simulink model "trng_controller_emu"  (R2024a)
settings: Solver=FixedStepAuto  StartTime=0.0  StopTime=250  FixedStep=20e-3  RelTol=1e-3
model workspace (MAT data in the model file):
  Ki = 10
  Kp = 100
undefined symbols (not defined in the file or in its folder): DiscIntNeverNeededParam
libraries: dspstat3 x3
settings Model: Creator=manik  LastModifiedBy=manik

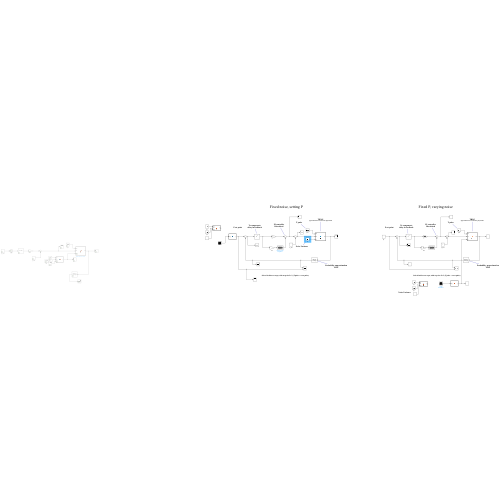
[thumbnail: Simulink's stored preview of the top-level diagram]
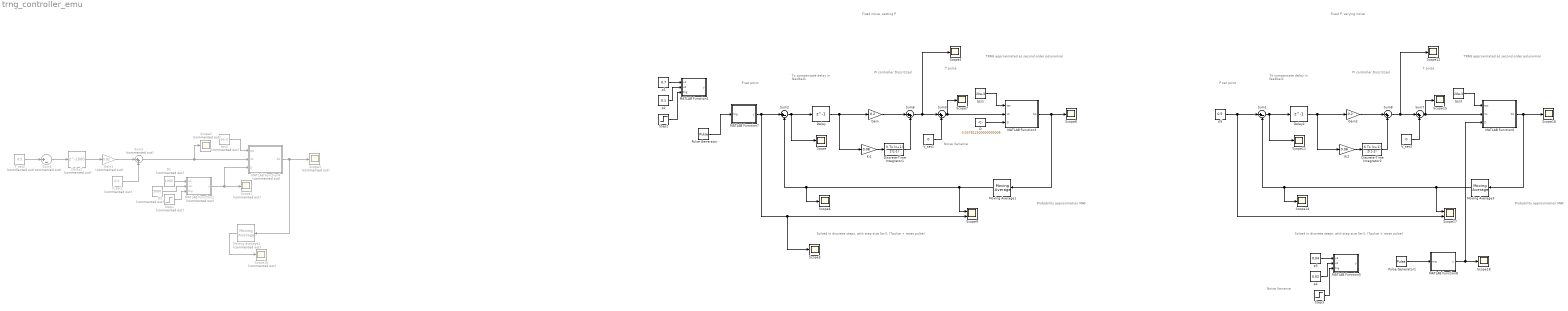
== system trng_controller_emu ==
  note: Fixed P, varying noise
  note: To compensate
      | delay in feedback
  note: PI controller
      | Discritized
  note: TRNG
      | approximated as second order polynomial
  note: T pulse
  note: Noise Variance
  note: Probability approximation
      | MAF
  note: Solved in discrete steps, with step size 5e-3, (Tpulse + reset pulse)
  note: P set point
  note: To compensate
      | delay in feedback
  note: PI controller
      | Discritized
  note: T pulse
  note: Probability approximation
      | MAF
  note: TRNG
      | approximated as second order polynomial
  note: Solved in discrete steps, with step size 5e-3, (Tpulse + reset pulse)
  note: P set point
  note: Fixed noise, setting P
  note: Noise Variance
  D : Constant  Value=0.037812500000000006
  D1 : Constant  Commented=on  Value=1000
  D2 : Constant  Commented=on  Value=5000
  Delay : Delay  DelayLength=1  InputProcessing=Columns as channels (frame based)  SampleTime=20e-3
  Delay1 : Delay  Commented=on  DelayLength=1000  InputProcessing=Columns as channels (frame based)
  Delay2 : Delay  DelayLength=1  InputProcessing=Columns as channels (frame based)  SampleTime=20e-3
  Discrete-Time Integrator1 : DiscreteIntegrator  IntegratorMethod=Integration: Trapezoidal  SampleTime=20e-3  ICPrevOutput=DiscIntNeverNeededParam  ICPrevScaledInput=DiscIntNeverNeededParam
  Discrete-Time Integrator2 : DiscreteIntegrator  IntegratorMethod=Integration: Trapezoidal  SampleTime=20e-3  ICPrevOutput=DiscIntNeverNeededParam  ICPrevScaledInput=DiscIntNeverNeededParam
  Gain : Gain  Gain=0.2
  Gain1 : Gain  Commented=on  Gain=0.02
  Gain2 : Gain  Gain=0.2
  Ki1 : Gain  Gain=0.08
  Ki2 : Gain  Gain=0.08
  MATLAB Function1 : MATLAB Function  TreatAsAtomicUnit=on
  MATLAB Function2 : MATLAB Function  Commented=on  TreatAsAtomicUnit=on
  MATLAB Function3 : MATLAB Function  TreatAsAtomicUnit=on
  MATLAB Function4 : MATLAB Function  Commented=on  TreatAsAtomicUnit=on
  MATLAB Function5 : MATLAB Function  TreatAsAtomicUnit=on
  MATLAB Function6 : MATLAB Function  TreatAsAtomicUnit=on
  MATLAB Function7 : MATLAB Function  TreatAsAtomicUnit=on
  MATLAB Function8 : MATLAB Function  TreatAsAtomicUnit=on
  Moving Average1 : dspstat3/Moving Average  Method=Sliding window  ForgettingFactorPort=off  SpecifyWindowLength=on  WindowLength=100  OverlapLength=99  AllowArbitraryInputLength=off  ForgettingFactor=0.9  SimulateUsing=Interpreted execution
  Moving Average2 : dspstat3/Moving Average  Commented=on  Method=Sliding window  ForgettingFactorPort=off  SpecifyWindowLength=on  WindowLength=1000  OverlapLength=999  AllowArbitraryInputLength=off  ForgettingFactor=0.9  SimulateUsing=Interpreted execution
  Moving Average3 : dspstat3/Moving Average  Method=Sliding window  ForgettingFactorPort=off  SpecifyWindowLength=on  WindowLength=100  OverlapLength=99  AllowArbitraryInputLength=off  ForgettingFactor=0.9  SimulateUsing=Interpreted execution
  P_set2 : Constant  Commented=on  Value=0.5
  Pulse Generator : DiscretePulseGenerator  PulseType=Time based  Period=50  PulseWidth=5
  Pulse Generator1 : DiscretePulseGenerator  PulseType=Time based  Period=50
  Scope{,4..8,11..12,14..16,18} (12 alike) : Scope
  Scope{1..3,10} (4 alike) : Scope  Commented=on
  Scope17 : Scope  NumInputPorts=2
  Scope9 : Scope  NumInputPorts=2
  Step1 : Step  Commented=on  Time=25  SampleTime=0
  Step2 : Step  Time=50  SampleTime=0
  Step3 : Step  Time=50  SampleTime=0
  Sum1 : Sum  Inputs=|+-
  Sum2 : Sum  Inputs=|+-
  Sum{3,6..8} (4 alike) : Sum  Inputs=|++
  Sum4 : Sum  Commented=on  Inputs=|+-
  Sum5 : Sum  Commented=on  Inputs=|++
  V_set1 : Constant  Value=0
  V_set2 : Constant  Commented=on  Value=0.2
  V_set3 : Constant  Value=0
  p1 : Constant  Value=0.7
  p2 : Constant  Value=0.1
  p3 : Constant  Value=0.04
  p4 : Constant  Value=0.02
  p5 : Constant  Value=0.5
  tps1 : Constant  Value=20e-3
  tps2 : Constant  Commented=on  Value=1e-3
  tps3 : Constant  Value=20e-3
  wires:
  V_set1/1 -> Sum3/2
  tps1/1 -> MATLAB Function3/1(tps)
  Sum3/1 -> Scope7/1, MATLAB Function3/2(Vs)
  MATLAB Function3/1(bit) -> Scope8/1, Moving Average1/1
  Moving Average1/1 -> Scope6/1, Sum2/2, Scope9/1
  Sum2/1 -> Scope/1, Delay/1
  Delay/1 -> Ki1/1, Gain/1
  tps2/1 -> MATLAB Function4/1(tps)
  MATLAB Function4/1(bit) -> Scope3/1, Moving Average2/1
  D1/1 -> MATLAB Function2/1(u1)
  MATLAB Function2/1(y) -> MATLAB Function4/3(D), Scope1/1
  Sum5/1 -> Scope2/1, MATLAB Function4/2(Vs)
  Step1/1 -> MATLAB Function2/3(trig)
  D2/1 -> MATLAB Function2/2(u2)
  Moving Average2/1 -> Scope10/1
  V_set2/1 -> Sum5/2
  Delay1/1 -> Gain1/1
  Sum4/1 -> Delay1/1
  Gain1/1 -> Sum5/1
  P_set2/1 -> Sum4/1
  D/1 -> MATLAB Function3/3(D)
  Discrete-Time Integrator1/1 -> Sum6/2
  Ki1/1 -> Discrete-Time Integrator1/1
  Gain/1 -> Sum6/1
  Sum6/1 -> Scope4/1, Sum3/1
  MATLAB Function7/1(y) -> Scope5/1, Scope9/2, Sum2/1
  Sum7/1 -> Scope15/1, MATLAB Function6/2(Vs)
  Delay2/1 -> Ki2/1, Gain2/1
  Discrete-Time Integrator2/1 -> Sum8/2
  Ki2/1 -> Discrete-Time Integrator2/1
  Gain2/1 -> Sum8/1
  Sum8/1 -> Scope12/1, Sum7/1
  Moving Average3/1 -> Scope14/1, Sum1/2, Scope17/1
  V_set3/1 -> Sum7/2
  MATLAB Function6/1(bit) -> Scope16/1, Moving Average3/1
  tps3/1 -> MATLAB Function6/1(tps)
  MATLAB Function8/1(y) -> MATLAB Function6/3(D), Scope18/1
  Sum1/1 -> Scope11/1, Delay2/1
  p5/1 -> Scope17/2, Sum1/1
  p1/1 -> MATLAB Function1/1(u1)
  p2/1 -> MATLAB Function1/2(u2)
  Step2/1 -> MATLAB Function1/3(trig)
  Pulse Generator/1 -> MATLAB Function7/1(trig)
  p4/1 -> MATLAB Function5/2(u2)
  p3/1 -> MATLAB Function5/1(u1)
  Step3/1 -> MATLAB Function5/3(trig)
  Pulse Generator1/1 -> MATLAB Function8/1(trig)

== matlab function trng_controller_emu/MATLAB Function1 ==
  data: u1 input; y output; u2 input; trig input
function y = sw(u1, u2, trig)

if(trig == 0)
    y = u1;
else
    y = u2;
end

== matlab function trng_controller_emu/MATLAB Function2 ==
  data: u1 input; y output; u2 input; trig input
function y = sw(u1, u2, trig)

if(trig == 0)
    y = u1;
else
    y = u2;
end

== matlab function trng_controller_emu/MATLAB Function4 ==
  data: tps input; bit output; Vs input; D input
function bit = fcn(tps, Vs, D)
    % Constants
    alpha = -1e4;
    beta = 1e4;
    
    DU = 9705*Vs^2 - 15030*Vs + 2536;
    PA = 1.263*Vs^2 + 0.2756*Vs - 0.9846;
    PC = -1.064*Vs^2 - 0.7479*Vs - 0.01687;

    D2UA = alpha + 3*beta*PA^2; 
    D2UC = alpha + 3*beta*PC^2;

    rk = abs(D2UA*D2UC)^0.5/(2*pi)*exp(-DU/D);

    p = 1 - exp(-tps*rk);
    if (rand(1,1) < p)
        bit = 1;
    else
        bit = 0;
    end

== matlab function trng_controller_emu/MATLAB Function3 ==
  data: tps input; bit output; Vs input; D input
function bit = fcn(tps, Vs, D)
    % Constants
    alpha = -0.97;
    beta = 1.05;
    rho = 0.0002;

    DU = 1.05862612*Vs^2 - 1.0409353*Vs + 0.2249036;
    PA = -1.38128915*Vs^2 -0.39070735*Vs - 0.95680691;
    PC = 1.11335556*Vs^2 + 0.91301695*Vs + 0.00476575;

    D2UA = alpha + 3*beta*PA^2; 
    D2UC = alpha + 3*beta*PC^2;

    rk = abs(D2UA*D2UC)^0.5/(2*pi*rho)*exp(-DU/D);

    p = 1 - exp(-tps*rk);
    if (rand(1,1) < p)
        bit = 1;
    else
        bit = 0;
    end

== matlab function trng_controller_emu/MATLAB Function5 ==
  data: u1 input; y output; u2 input; trig input
function y = sw(u1, u2, trig)

if(trig == 0)
    y = u1;
else
    y = u2;
end

== matlab function trng_controller_emu/MATLAB Function6 ==
  data: tps input; bit output; Vs input; D input
function bit = fcn(tps, Vs, D)
    % Constants
    alpha = -0.97;
    beta = 1.05;
    rho = 0.0002;

    DU = 1.05862612*Vs^2 - 1.0409353*Vs + 0.2249036;
    PA = -1.38128915*Vs^2 -0.39070735*Vs - 0.95680691;
    PC = 1.11335556*Vs^2 + 0.91301695*Vs + 0.00476575;

    D2UA = alpha + 3*beta*PA^2; 
    D2UC = alpha + 3*beta*PC^2;

    rk = abs(D2UA*D2UC)^0.5/(2*pi*rho)*exp(-DU/D);

    p = 1 - exp(-tps*rk);
    if (rand(1,1) < p)
        bit = 1;
    else
        bit = 0;
    end

== matlab function trng_controller_emu/MATLAB Function7 ==
  data: y output; trig input
function y = sw(trig)
    persistent trg_prev y_prev;

    if isempty(trg_prev)
        trg_prev = trig;
        y_prev = 0.5;   % Initial value
    end

    % Detect edge (change)
    if (trig - trg_prev) > 0.9
        y_prev = rand();  % Generate new value only once per edge
    end

    trg_prev = trig;  % Update for next comparison
    y = y_prev;       % Hold the value
end

== matlab function trng_controller_emu/MATLAB Function8 ==
  data: y output; trig input
function y = sw(trig)

    persistent trg_prev y_prev;

    if isempty(trg_prev)
        trg_prev = trig;
        y_prev = 0.03;   % Initial value
    end

    % Detect edge (change)
    if (trig - trg_prev) > 0.9
        y_prev = 0.025 + (0.04 - 0.025) * rand();
    end

    trg_prev = trig;  % Update for next comparison
    y = y_prev;       % Hold the value
end
